simulink model "Case3_IEEE39_UGFLandGFM_2022b"  (R2022b)
settings: Solver=VariableStepAuto  StartTime=0.0  StopTime=30  RelTol=1e-3
InitFcn:
  | IEEE39data_UGFLandGFM;
undefined symbols (not defined in the file): Fref, IBR, line, Sbase, SG, UGFML, Vbase
libraries: spsThreePhaseVIMeasurementLib x66, spsThreePhasePISectionLineLib x35, spsPLL3phLib x25, spsControlledVoltageSourceLib x21, spsThreePhaseParallelRLCLoadLib x21, powerlib_extras x20, spsGroundLib x20, spsMeanLib x20, spsRMSLib x15, spsabctodq0Lib x11, spsThreePhaseSeriesRLCBranchLib x10, slpidlib x10
(part 3 of 5)

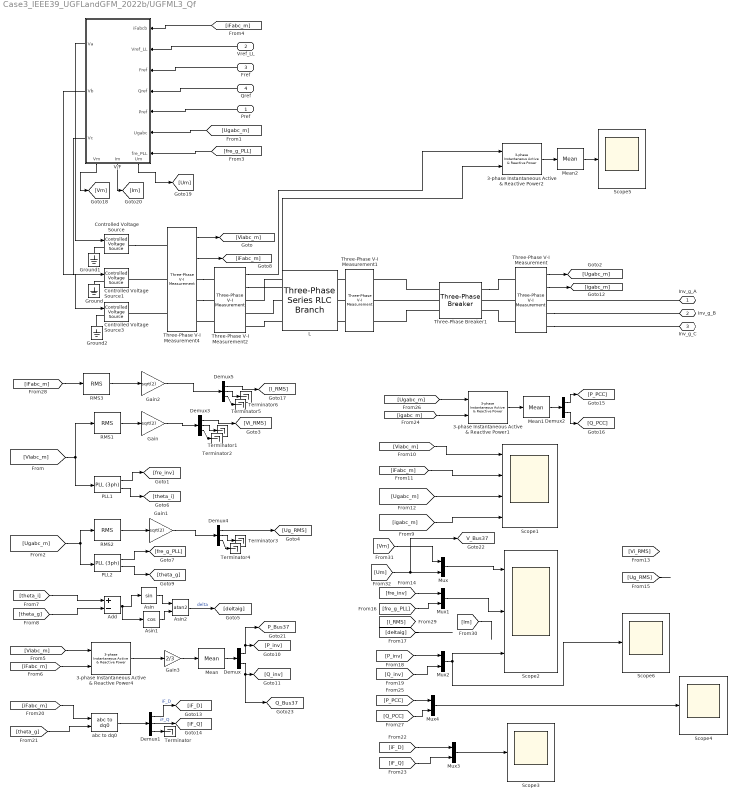
== system Case3_IEEE39_UGFLandGFM_2022b/UGFML3_Qf ==
  Pref : Inport
  Vref_LL : Inport  Port=2
  Fref : Inport  Port=3
  Qref : Inport  Port=4
  3-phase Instantaneous Active & Reactive Power1 : powerlib_extras/Measurements/3-phase  Instantaneous  Active & Reactive Power
  3-phase Instantaneous Active & Reactive Power2 : powerlib_extras/Measurements/3-phase  Instantaneous  Active & Reactive Power
  3-phase Instantaneous Active & Reactive Power4 : powerlib_extras/Measurements/3-phase  Instantaneous  Active & Reactive Power
  Add : Sum  Inputs=+-
  Asin : Trigonometry
  Asin1 : Trigonometry  Operator=cos
  Asin2 : Trigonometry  Operator=atan2
  Controlled Voltage Source : spsControlledVoltageSourceLib/Controlled Voltage Source  Initialize=on  Source_Type=DC  Amplitude=300  Phase=0  Frequency=60  Measurements=None
  Controlled Voltage Source1 : spsControlledVoltageSourceLib/Controlled Voltage Source  Initialize=on  Source_Type=DC  Amplitude=300  Phase=-120  Frequency=60  Measurements=None
  Controlled Voltage Source3 : spsControlledVoltageSourceLib/Controlled Voltage Source  Initialize=on  Source_Type=DC  Amplitude=300  Phase=120  Frequency=60  Measurements=None
  Demux : Demux  Outputs=2
  Demux{1,3..5} (4 alike) : Demux  Outputs=3
  Demux2 : Demux  Outputs=2
  Gain : Gain  Gain=sqrt(2)
  Gain1 : Gain  Gain=sqrt(2)
  Gain2 : Gain  Gain=sqrt(2)
  Gain3 : Gain  Gain=2/3
  Ground : spsGroundLib/Ground  LConnTagsString=a
  Ground1 : spsGroundLib/Ground  LConnTagsString=a
  Ground2 : spsGroundLib/Ground  LConnTagsString=a
  L : spsThreePhaseSeriesRLCBranchLib/Three-Phase Series RLC Branch  LConnTagsString=A|B|C  RConnTagsString=A|B|C  BranchType=RL  Resistance=0.01*Vbase^2/Sbase  Inductance=0.05*(Vbase^2/Sbase/377)  Capacitance=1.0  Measurements=None
  Mean : spsMeanLib/Mean  Freq=60  Vinit=0  Ts=5e-4
  Mean1 : spsMeanLib/Mean  Freq=60  Vinit=0  Ts=1e-4
  Mean2 : spsMeanLib/Mean  Freq=60  Vinit=0  Ts=5e-4
  Mux{,1..4} (5 alike) : Mux  Inputs=2
  PLL1 : spsPLL3phLib/PLL (3ph)  Fmin=35  Par_Init=[0, 60]  ParK=[180, 3200, 1]  TcD=1e-4  MaxRateChangeFreq=12  FilterCutOffFreq=25  Ts=1e-5  AGC=on
  PLL2 : spsPLL3phLib/PLL (3ph)  Fmin=35  Par_Init=[0, 60]  ParK=[180, 3200, 1]  TcD=1e-4  MaxRateChangeFreq=12  FilterCutOffFreq=25  Ts=1e-5  AGC=on
  RMS1 : spsRMSLib/RMS  TrueRMS=on  Freq=60  RMSInit=1  Ts=1e-4
  RMS2 : spsRMSLib/RMS  TrueRMS=on  Freq=60  RMSInit=1  Ts=1e-4
  RMS3 : spsRMSLib/RMS  TrueRMS=on  Freq=60  RMSInit=1  Ts=5e-4
  Scope1 : Scope  NumInputPorts=4
  Scope2 : Scope  NumInputPorts=3
  Scope{3..6} (4 alike) : Scope
  Terminator{,1..6} (7 alike) : Terminator
  Three-Phase V-I Measurement : spsThreePhaseVIMeasurementLib/Three-Phase V-I Measurement  VoltageMeasurement=phase-to-ground  SetLabelV=off  LabelV=Vabc  Vpu=on  VpuLL=off  CurrentMeasurement=yes  SetLabelI=off  LabelI=Iabc  Ipu=on  Pbase=Sbase  Vbase=Vbase  OutputType=Complex  PhasorSimulation=off  PSBequivalent=0
  Three-Phase V-I Measurement1 : spsThreePhaseVIMeasurementLib/Three-Phase V-I Measurement  VoltageMeasurement=no  SetLabelV=off  LabelV=Vabc  Vpu=off  VpuLL=off  CurrentMeasurement=no  SetLabelI=off  LabelI=Iabc  Ipu=off  Pbase=1e5  Vbase=380  OutputType=Complex  PhasorSimulation=off  PSBequivalent=0
  Three-Phase V-I Measurement2 : spsThreePhaseVIMeasurementLib/Three-Phase V-I Measurement  VoltageMeasurement=phase-to-ground  SetLabelV=off  LabelV=Vabc  Vpu=off  VpuLL=off  CurrentMeasurement=yes  SetLabelI=off  LabelI=Iabc  Ipu=off  Pbase=Sbase  Vbase=Vbase  OutputType=Complex  PhasorSimulation=off  PSBequivalent=0
  Three-Phase V-I Measurement4 : spsThreePhaseVIMeasurementLib/Three-Phase V-I Measurement  VoltageMeasurement=phase-to-ground  SetLabelV=off  LabelV=u  Vpu=on  VpuLL=off  CurrentMeasurement=yes  SetLabelI=off  LabelI=iFabcp3  Ipu=on  Pbase=Sbase  Vbase=Vbase  OutputType=Complex  PhasorSimulation=off  PSBequivalent=0
  Three-Phase Breaker1 : spsThreePhaseBreakerLib/Three-Phase Breaker  InitialState=open  SwitchA=on  SwitchB=on  SwitchC=on  SwitchTimes=[0.1]  External=off  BreakerResistance=0.0001  SnubberResistance=1e8  SnubberCapacitance=inf  Measurements=None
  V/F : Subsystem
      settings: PortSchema="{\"entries\":[{\"content\":{\"sides\":[{\"content\":{\"connectorIds\":[\"In1\",\"In2\",\"In3\",\"In4\",\"In5\",\"In6\",\"In7\"]},\"type\":\"ConnectorPlacement.EquallySpacedRectSide\",\"uuid\":\"ccc7dc11-36db-4369-953c-0655fd1e2442\"},{\"content\":{\"connectorIds\":[\"Out1\",\"Out2\",\"Out3\"],\"side\":\"RIGHT\"},\"type\":\"ConnectorPlacement.EquallySpacedRectSide\",\"uuid\":\"5735cf9b-d8e4-4bce-b2db-12738d0d9e4d\"},{\"content\":{\"side\":\"TOP\"},\"type\":\"ConnectorPlacement.EquallySpacedRectSide\",\"uuid\":\"e010782d-2644-4ebf-978f-8395ad947d0e\"},{\"content\":{\"connectorIds\":[\"Out4\",\"Out5\",\"Out6\"],\"side\":\"BOTTOM\"},\"type\":\"ConnectorPlacement.EquallySpacedRectSide\",\"uuid\":\"5965ef6f-6121-4d63-9a5a-1f7a3d153058\"}]},\"type\":\"ConnectorPlacement.EquallySpacedConnector\",\"uuid\":\"be33ea6e-20ef-4fc3-81eb-341d11cc9c18\"}],\"packageUris\":[\"http://schema.mathworks.com/mf0/Connector/R2020b\"],\"version\":\"1.0\"}"
  abc to dq0 : spsabctodq0Lib/abc to dq0  Alignment=90 degrees behind phase A axis
  Inv_g_A : PMIOPort  Side=Right
  Inv_g_B : PMIOPort  Port=2  Side=Right
  Inv_g_C : PMIOPort  Port=3  Side=Right
  tag scope: P_Bus37=global, Q_Bus37=global, V_Bus37=global
  wires:
  Three-Phase V-I Measurement/1 -> [Ugabc_m]
  Vref_LL/1 -> V/F/2(Vref_LL)
  V/F/2(Vb) -> Controlled Voltage Source1/1
  V/F/3(Vc) -> Controlled Voltage Source3/1
  Pref/1 -> V/F/5(Pref)
  Qref/1 -> V/F/4(Qref)
  Fref/1 -> V/F/3(Fref)
  RMS1/1 -> Gain/1
  Three-Phase V-I Measurement4/1 -> [Viabc_m]
  [Viabc_m] -> RMS1/1, PLL1/1
  PLL1/2 -> [theta_i]
  PLL1/1 -> [fre_inv]
  [Ugabc_m] -> V/F/6(Ugabc)
  [Ugabc_m] -> PLL2/1, RMS2/1
  RMS2/1 -> Gain1/1
  PLL2/2 -> [theta_g]
  PLL2/1 -> [fre_g_PLL]
  Three-Phase V-I Measurement4/2 -> [iFabc_m]
  [iFabc_m] -> V/F/1(iFabcb)
  [Viabc_m] -> 3-phase Instantaneous Active & Reactive Power4/1
  [iFabc_m] -> 3-phase Instantaneous Active & Reactive Power4/2
  Mean/1 -> Demux/1
  Demux/1 -> [P_Bus37], [P_inv]
  Demux/2 -> [Q_Bus37], [Q_inv]
  Three-Phase V-I Measurement/2 -> [igabc_m]
  [Viabc_m] -> Scope1/1
  [iFabc_m] -> Scope1/2
  [Ugabc_m] -> Scope1/3
  [igabc_m] -> Scope1/4
  [fre_inv] -> Mux1/1
  [Ug_RMS] -> ?
  Mux/1 -> Scope2/1
  [fre_g_PLL] -> Mux1/2
  Mux1/1 -> Scope2/2
  [deltaig] -> ?
  [P_inv] -> Mux2/1
  [Q_inv] -> Mux2/2
  Mux2/1 -> Scope2/3, Scope6/1
  Gain/1 -> Demux3/1
  [fre_g_PLL] -> V/F/7(fre_PLL)
  [theta_i] -> Add/1
  Add/1 -> Asin/1, Asin1/1
  [theta_g] -> Add/2
  Asin/1 -> Asin2/1
  Asin1/1 -> Asin2/2
  Asin2/1 -> [deltaig]  "delta"
  [iFabc_m] -> abc to dq0/1
  [theta_g] -> abc to dq0/2
  abc to dq0/1 -> Demux1/1
  Demux1/3 -> Terminator/1
  Demux1/1 -> [iF_D]  "iF_D"
  Demux1/2 -> [iF_Q]  "iF_Q"
  [iF_D] -> Mux3/1
  [iF_Q] -> Mux3/2
  Mux3/1 -> Scope3/1
  V/F/1(Va) -> Controlled Voltage Source/1
  Demux2/2 -> [Q_PCC]
  [Ugabc_m] -> 3-phase Instantaneous Active & Reactive Power1/1
  [igabc_m] -> 3-phase Instantaneous Active & Reactive Power1/2
  Mean1/1 -> Demux2/1
  Demux2/1 -> [P_PCC]
  3-phase Instantaneous Active & Reactive Power1/1 -> Mean1/1
  [P_PCC] -> Mux4/1
  [Q_PCC] -> Mux4/2
  Mux4/1 -> Scope4/1
  Demux3/1 -> [Vi_RMS]
  Demux3/2 -> Terminator1/1
  Demux3/3 -> Terminator2/1
  Demux4/3 -> Terminator4/1
  Demux4/1 -> [Ug_RMS]
  Demux4/2 -> Terminator3/1
  Gain1/1 -> Demux4/1
  [iFabc_m] -> RMS3/1
  RMS3/1 -> Gain2/1
  Demux5/3 -> Terminator6/1
  Demux5/1 -> [I_RMS]
  Demux5/2 -> Terminator5/1
  Gain2/1 -> Demux5/1
  Three-Phase V-I Measurement2/1 -> 3-phase Instantaneous Active & Reactive Power2/1
  Mean2/1 -> Scope5/1
  Three-Phase V-I Measurement2/2 -> 3-phase Instantaneous Active & Reactive Power2/2
  3-phase Instantaneous Active & Reactive Power2/1 -> Mean2/1
  Gain3/1 -> Mean/1
  3-phase Instantaneous Active & Reactive Power4/1 -> Gain3/1
  [Vm] -> Mux/1
  [Um] -> [V_Bus37], Mux/2
  [Im] -> ?
  V/F/5(Im) -> [Im]
  V/F/6(Vm) -> [Vm]
  V/F/4(Um) -> [Um]
  connections:
  Three-Phase V-I Measurement/RConn2 -- Inv_g_B/RConn1
  Three-Phase V-I Measurement4/LConn2 -- Controlled Voltage Source1/RConn1
  Controlled Voltage Source/RConn1 -- Three-Phase V-I Measurement4/LConn1
  Three-Phase V-I Measurement4/LConn3 -- Controlled Voltage Source3/RConn1
  Three-Phase Breaker1/LConn3 -- Three-Phase V-I Measurement1/RConn3
  Three-Phase V-I Measurement/RConn3 -- Inv_g_C/RConn1
  Inv_g_A/RConn1 -- Three-Phase V-I Measurement/RConn1
  Three-Phase V-I Measurement4/RConn1 -- Three-Phase V-I Measurement2/LConn1
  Three-Phase V-I Measurement4/RConn2 -- Three-Phase V-I Measurement2/LConn2
  Three-Phase V-I Measurement2/LConn3 -- Three-Phase V-I Measurement4/RConn3
  Controlled Voltage Source1/LConn1 -- Ground/LConn1
  Three-Phase Breaker1/LConn2 -- Three-Phase V-I Measurement1/RConn2
  Three-Phase Breaker1/LConn1 -- Three-Phase V-I Measurement1/RConn1
  Three-Phase V-I Measurement1/LConn1 -- L/RConn1
  Three-Phase V-I Measurement1/LConn2 -- L/RConn2
  Three-Phase V-I Measurement1/LConn3 -- L/RConn3
  Controlled Voltage Source/LConn1 -- Ground1/LConn1
  Controlled Voltage Source3/LConn1 -- Ground2/LConn1
  Three-Phase Breaker1/RConn1 -- Three-Phase V-I Measurement/LConn1
  Three-Phase V-I Measurement/LConn2 -- Three-Phase Breaker1/RConn2
  Three-Phase V-I Measurement/LConn3 -- Three-Phase Breaker1/RConn3
  L/LConn1 -- Three-Phase V-I Measurement2/RConn1
  L/LConn2 -- Three-Phase V-I Measurement2/RConn2
  L/LConn3 -- Three-Phase V-I Measurement2/RConn3

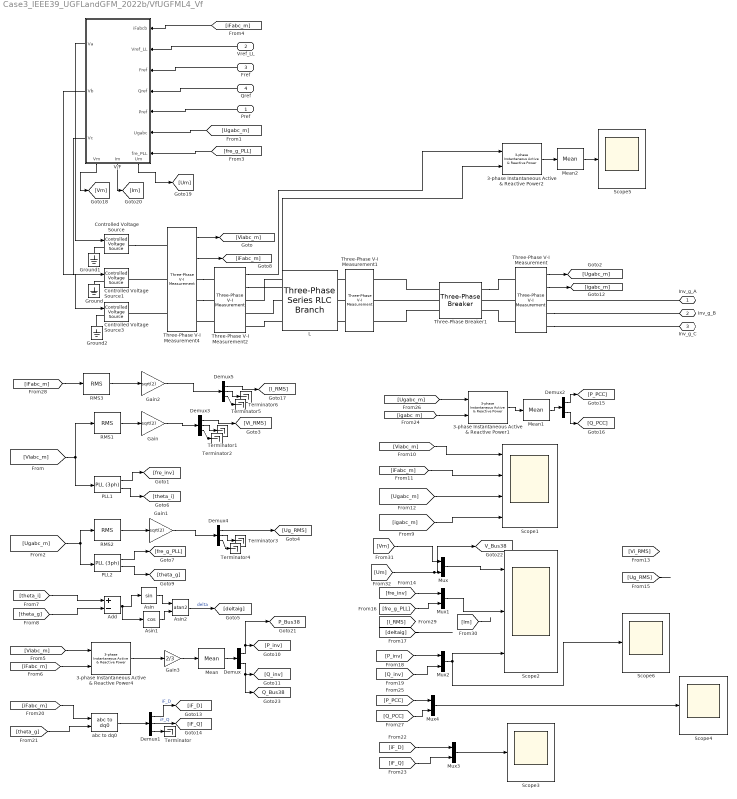
== system Case3_IEEE39_UGFLandGFM_2022b/VfUGFML4_Vf ==
  Pref : Inport
  Vref_LL : Inport  Port=2
  Fref : Inport  Port=3
  Qref : Inport  Port=4
  3-phase Instantaneous Active & Reactive Power1 : powerlib_extras/Measurements/3-phase  Instantaneous  Active & Reactive Power
  3-phase Instantaneous Active & Reactive Power2 : powerlib_extras/Measurements/3-phase  Instantaneous  Active & Reactive Power
  3-phase Instantaneous Active & Reactive Power4 : powerlib_extras/Measurements/3-phase  Instantaneous  Active & Reactive Power
  Add : Sum  Inputs=+-
  Asin : Trigonometry
  Asin1 : Trigonometry  Operator=cos
  Asin2 : Trigonometry  Operator=atan2
  Controlled Voltage Source : spsControlledVoltageSourceLib/Controlled Voltage Source  Initialize=on  Source_Type=DC  Amplitude=300  Phase=0  Frequency=60  Measurements=None
  Controlled Voltage Source1 : spsControlledVoltageSourceLib/Controlled Voltage Source  Initialize=on  Source_Type=DC  Amplitude=300  Phase=-120  Frequency=60  Measurements=None
  Controlled Voltage Source3 : spsControlledVoltageSourceLib/Controlled Voltage Source  Initialize=on  Source_Type=DC  Amplitude=300  Phase=120  Frequency=60  Measurements=None
  Demux : Demux  Outputs=2
  Demux{1,3..5} (4 alike) : Demux  Outputs=3
  Demux2 : Demux  Outputs=2
  Gain : Gain  Gain=sqrt(2)
  Gain1 : Gain  Gain=sqrt(2)
  Gain2 : Gain  Gain=sqrt(2)
  Gain3 : Gain  Gain=2/3
  Ground : spsGroundLib/Ground  LConnTagsString=a
  Ground1 : spsGroundLib/Ground  LConnTagsString=a
  Ground2 : spsGroundLib/Ground  LConnTagsString=a
  L : spsThreePhaseSeriesRLCBranchLib/Three-Phase Series RLC Branch  LConnTagsString=A|B|C  RConnTagsString=A|B|C  BranchType=RL  Resistance=0.01*Vbase^2/Sbase  Inductance=0.05*(Vbase^2/Sbase/377)  Capacitance=1.0  Measurements=None
  Mean : spsMeanLib/Mean  Freq=60  Vinit=0  Ts=5e-4
  Mean1 : spsMeanLib/Mean  Freq=60  Vinit=0  Ts=1e-4
  Mean2 : spsMeanLib/Mean  Freq=60  Vinit=0  Ts=5e-4
  Mux{,1..4} (5 alike) : Mux  Inputs=2
  PLL1 : spsPLL3phLib/PLL (3ph)  Fmin=35  Par_Init=[0, 60]  ParK=[180, 3200, 1]  TcD=1e-4  MaxRateChangeFreq=12  FilterCutOffFreq=25  Ts=1e-5  AGC=on
  PLL2 : spsPLL3phLib/PLL (3ph)  Fmin=35  Par_Init=[0, 60]  ParK=[180, 3200, 1]  TcD=1e-4  MaxRateChangeFreq=12  FilterCutOffFreq=25  Ts=1e-5  AGC=on
  RMS1 : spsRMSLib/RMS  TrueRMS=on  Freq=60  RMSInit=1  Ts=1e-4
  RMS2 : spsRMSLib/RMS  TrueRMS=on  Freq=60  RMSInit=1  Ts=1e-4
  RMS3 : spsRMSLib/RMS  TrueRMS=on  Freq=60  RMSInit=1  Ts=5e-4
  Scope1 : Scope  NumInputPorts=4
  Scope2 : Scope  NumInputPorts=3
  Scope{3..6} (4 alike) : Scope
  Terminator{,1..6} (7 alike) : Terminator
  Three-Phase V-I Measurement : spsThreePhaseVIMeasurementLib/Three-Phase V-I Measurement  VoltageMeasurement=phase-to-ground  SetLabelV=off  LabelV=Vabc  Vpu=on  VpuLL=off  CurrentMeasurement=yes  SetLabelI=off  LabelI=Iabc  Ipu=on  Pbase=Sbase  Vbase=Vbase  OutputType=Complex  PhasorSimulation=off  PSBequivalent=0
  Three-Phase V-I Measurement1 : spsThreePhaseVIMeasurementLib/Three-Phase V-I Measurement  VoltageMeasurement=no  SetLabelV=off  LabelV=Vabc  Vpu=off  VpuLL=off  CurrentMeasurement=no  SetLabelI=off  LabelI=Iabc  Ipu=off  Pbase=1e5  Vbase=380  OutputType=Complex  PhasorSimulation=off  PSBequivalent=0
  Three-Phase V-I Measurement2 : spsThreePhaseVIMeasurementLib/Three-Phase V-I Measurement  VoltageMeasurement=phase-to-ground  SetLabelV=off  LabelV=Vabc  Vpu=off  VpuLL=off  CurrentMeasurement=yes  SetLabelI=off  LabelI=Iabc  Ipu=off  Pbase=Sbase  Vbase=Vbase  OutputType=Complex  PhasorSimulation=off  PSBequivalent=0
  Three-Phase V-I Measurement4 : spsThreePhaseVIMeasurementLib/Three-Phase V-I Measurement  VoltageMeasurement=phase-to-ground  SetLabelV=off  LabelV=u  Vpu=on  VpuLL=off  CurrentMeasurement=yes  SetLabelI=off  LabelI=iFabcp3  Ipu=on  Pbase=Sbase  Vbase=Vbase  OutputType=Complex  PhasorSimulation=off  PSBequivalent=0
  Three-Phase Breaker1 : spsThreePhaseBreakerLib/Three-Phase Breaker  InitialState=open  SwitchA=on  SwitchB=on  SwitchC=on  SwitchTimes=[0.1]  External=off  BreakerResistance=0.0001  SnubberResistance=1e8  SnubberCapacitance=inf  Measurements=None
  V/F : Subsystem
      settings: PortSchema="{\"entries\":[{\"content\":{\"sides\":[{\"content\":{\"connectorIds\":[\"In1\",\"In2\",\"In3\",\"In4\",\"In5\",\"In6\",\"In7\"]},\"type\":\"ConnectorPlacement.EquallySpacedRectSide\",\"uuid\":\"ccc7dc11-36db-4369-953c-0655fd1e2442\"},{\"content\":{\"connectorIds\":[\"Out1\",\"Out2\",\"Out3\"],\"side\":\"RIGHT\"},\"type\":\"ConnectorPlacement.EquallySpacedRectSide\",\"uuid\":\"5735cf9b-d8e4-4bce-b2db-12738d0d9e4d\"},{\"content\":{\"side\":\"TOP\"},\"type\":\"ConnectorPlacement.EquallySpacedRectSide\",\"uuid\":\"e010782d-2644-4ebf-978f-8395ad947d0e\"},{\"content\":{\"connectorIds\":[\"Out4\",\"Out5\",\"Out6\"],\"side\":\"BOTTOM\"},\"type\":\"ConnectorPlacement.EquallySpacedRectSide\",\"uuid\":\"5965ef6f-6121-4d63-9a5a-1f7a3d153058\"}]},\"type\":\"ConnectorPlacement.EquallySpacedConnector\",\"uuid\":\"be33ea6e-20ef-4fc3-81eb-341d11cc9c18\"}],\"packageUris\":[\"http://schema.mathworks.com/mf0/Connector/R2020b\"],\"version\":\"1.0\"}"
  abc to dq0 : spsabctodq0Lib/abc to dq0  Alignment=90 degrees behind phase A axis
  Inv_g_A : PMIOPort  Side=Right
  Inv_g_B : PMIOPort  Port=2  Side=Right
  Inv_g_C : PMIOPort  Port=3  Side=Right
  tag scope: P_Bus38=global, Q_Bus38=global, V_Bus38=global
  wires:
  Three-Phase V-I Measurement/1 -> [Ugabc_m]
  Vref_LL/1 -> V/F/2(Vref_LL)
  V/F/2(Vb) -> Controlled Voltage Source1/1
  V/F/3(Vc) -> Controlled Voltage Source3/1
  Pref/1 -> V/F/5(Pref)
  Qref/1 -> V/F/4(Qref)
  Fref/1 -> V/F/3(Fref)
  RMS1/1 -> Gain/1
  Three-Phase V-I Measurement4/1 -> [Viabc_m]
  [Viabc_m] -> RMS1/1, PLL1/1
  PLL1/2 -> [theta_i]
  PLL1/1 -> [fre_inv]
  [Ugabc_m] -> V/F/6(Ugabc)
  [Ugabc_m] -> PLL2/1, RMS2/1
  RMS2/1 -> Gain1/1
  PLL2/2 -> [theta_g]
  PLL2/1 -> [fre_g_PLL]
  Three-Phase V-I Measurement4/2 -> [iFabc_m]
  [iFabc_m] -> V/F/1(iFabcb)
  [Viabc_m] -> 3-phase Instantaneous Active & Reactive Power4/1
  [iFabc_m] -> 3-phase Instantaneous Active & Reactive Power4/2
  Mean/1 -> Demux/1
  Demux/1 -> [P_Bus38], [P_inv]
  Demux/2 -> [Q_Bus38], [Q_inv]
  Three-Phase V-I Measurement/2 -> [igabc_m]
  [Viabc_m] -> Scope1/1
  [iFabc_m] -> Scope1/2
  [Ugabc_m] -> Scope1/3
  [igabc_m] -> Scope1/4
  [fre_inv] -> Mux1/1
  [Ug_RMS] -> ?
  Mux/1 -> Scope2/1
  [fre_g_PLL] -> Mux1/2
  Mux1/1 -> Scope2/2
  [deltaig] -> ?
  [P_inv] -> Mux2/1
  [Q_inv] -> Mux2/2
  Mux2/1 -> Scope2/3, Scope6/1
  Gain/1 -> Demux3/1
  [fre_g_PLL] -> V/F/7(fre_PLL)
  [theta_i] -> Add/1
  Add/1 -> Asin/1, Asin1/1
  [theta_g] -> Add/2
  Asin/1 -> Asin2/1
  Asin1/1 -> Asin2/2
  Asin2/1 -> [deltaig]  "delta"
  [iFabc_m] -> abc to dq0/1
  [theta_g] -> abc to dq0/2
  abc to dq0/1 -> Demux1/1
  Demux1/3 -> Terminator/1
  Demux1/1 -> [iF_D]  "iF_D"
  Demux1/2 -> [iF_Q]  "iF_Q"
  [iF_D] -> Mux3/1
  [iF_Q] -> Mux3/2
  Mux3/1 -> Scope3/1
  V/F/1(Va) -> Controlled Voltage Source/1
  Demux2/2 -> [Q_PCC]
  [Ugabc_m] -> 3-phase Instantaneous Active & Reactive Power1/1
  [igabc_m] -> 3-phase Instantaneous Active & Reactive Power1/2
  Mean1/1 -> Demux2/1
  Demux2/1 -> [P_PCC]
  3-phase Instantaneous Active & Reactive Power1/1 -> Mean1/1
  [P_PCC] -> Mux4/1
  [Q_PCC] -> Mux4/2
  Mux4/1 -> Scope4/1
  Demux3/1 -> [Vi_RMS]
  Demux3/2 -> Terminator1/1
  Demux3/3 -> Terminator2/1
  Demux4/3 -> Terminator4/1
  Demux4/1 -> [Ug_RMS]
  Demux4/2 -> Terminator3/1
  Gain1/1 -> Demux4/1
  [iFabc_m] -> RMS3/1
  RMS3/1 -> Gain2/1
  Demux5/3 -> Terminator6/1
  Demux5/1 -> [I_RMS]
  Demux5/2 -> Terminator5/1
  Gain2/1 -> Demux5/1
  Three-Phase V-I Measurement2/1 -> 3-phase Instantaneous Active & Reactive Power2/1
  Mean2/1 -> Scope5/1
  Three-Phase V-I Measurement2/2 -> 3-phase Instantaneous Active & Reactive Power2/2
  3-phase Instantaneous Active & Reactive Power2/1 -> Mean2/1
  Gain3/1 -> Mean/1
  3-phase Instantaneous Active & Reactive Power4/1 -> Gain3/1
  [Vm] -> Mux/1
  [Um] -> [V_Bus38], Mux/2
  [Im] -> ?
  V/F/5(Im) -> [Im]
  V/F/6(Vm) -> [Vm]
  V/F/4(Um) -> [Um]
  connections:
  Three-Phase V-I Measurement/RConn2 -- Inv_g_B/RConn1
  Three-Phase V-I Measurement4/LConn2 -- Controlled Voltage Source1/RConn1
  Controlled Voltage Source/RConn1 -- Three-Phase V-I Measurement4/LConn1
  Three-Phase V-I Measurement4/LConn3 -- Controlled Voltage Source3/RConn1
  Three-Phase Breaker1/LConn3 -- Three-Phase V-I Measurement1/RConn3
  Three-Phase V-I Measurement/RConn3 -- Inv_g_C/RConn1
  Inv_g_A/RConn1 -- Three-Phase V-I Measurement/RConn1
  Three-Phase V-I Measurement4/RConn1 -- Three-Phase V-I Measurement2/LConn1
  Three-Phase V-I Measurement4/RConn2 -- Three-Phase V-I Measurement2/LConn2
  Three-Phase V-I Measurement2/LConn3 -- Three-Phase V-I Measurement4/RConn3
  Controlled Voltage Source1/LConn1 -- Ground/LConn1
  Three-Phase Breaker1/LConn2 -- Three-Phase V-I Measurement1/RConn2
  Three-Phase Breaker1/LConn1 -- Three-Phase V-I Measurement1/RConn1
  Three-Phase V-I Measurement1/LConn1 -- L/RConn1
  Three-Phase V-I Measurement1/LConn2 -- L/RConn2
  Three-Phase V-I Measurement1/LConn3 -- L/RConn3
  Controlled Voltage Source/LConn1 -- Ground1/LConn1
  Controlled Voltage Source3/LConn1 -- Ground2/LConn1
  Three-Phase Breaker1/RConn1 -- Three-Phase V-I Measurement/LConn1
  Three-Phase V-I Measurement/LConn2 -- Three-Phase Breaker1/RConn2
  Three-Phase V-I Measurement/LConn3 -- Three-Phase Breaker1/RConn3
  L/LConn1 -- Three-Phase V-I Measurement2/RConn1
  L/LConn2 -- Three-Phase V-I Measurement2/RConn2
  L/LConn3 -- Three-Phase V-I Measurement2/RConn3

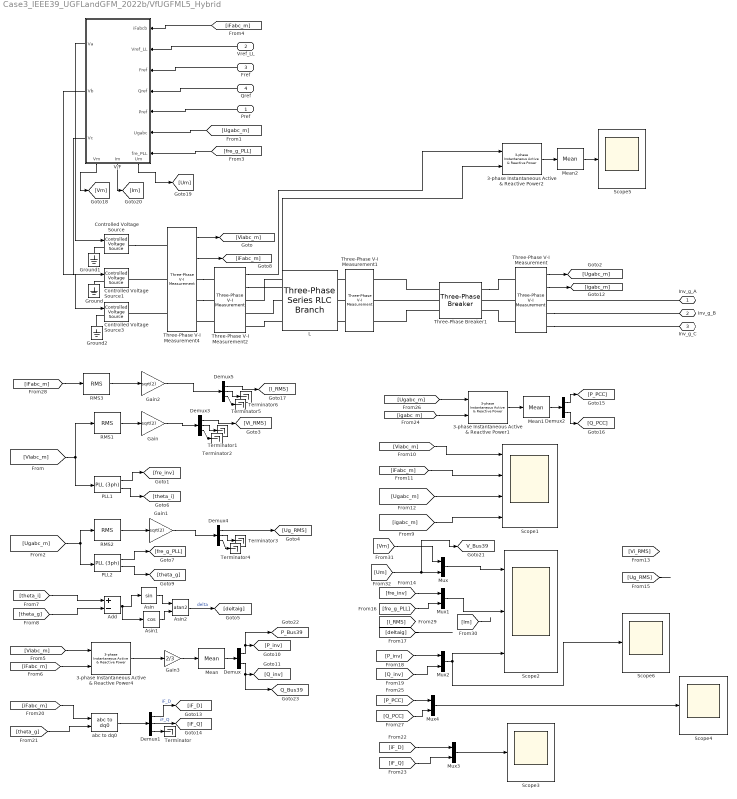
== system Case3_IEEE39_UGFLandGFM_2022b/VfUGFML5_Hybrid ==
  Pref : Inport
  Vref_LL : Inport  Port=2
  Fref : Inport  Port=3
  Qref : Inport  Port=4
  3-phase Instantaneous Active & Reactive Power1 : powerlib_extras/Measurements/3-phase  Instantaneous  Active & Reactive Power
  3-phase Instantaneous Active & Reactive Power2 : powerlib_extras/Measurements/3-phase  Instantaneous  Active & Reactive Power
  3-phase Instantaneous Active & Reactive Power4 : powerlib_extras/Measurements/3-phase  Instantaneous  Active & Reactive Power
  Add : Sum  Inputs=+-
  Asin : Trigonometry
  Asin1 : Trigonometry  Operator=cos
  Asin2 : Trigonometry  Operator=atan2
  Controlled Voltage Source : spsControlledVoltageSourceLib/Controlled Voltage Source  Initialize=on  Source_Type=DC  Amplitude=300  Phase=0  Frequency=60  Measurements=None
  Controlled Voltage Source1 : spsControlledVoltageSourceLib/Controlled Voltage Source  Initialize=on  Source_Type=DC  Amplitude=300  Phase=-120  Frequency=60  Measurements=None
  Controlled Voltage Source3 : spsControlledVoltageSourceLib/Controlled Voltage Source  Initialize=on  Source_Type=DC  Amplitude=300  Phase=120  Frequency=60  Measurements=None
  Demux : Demux  Outputs=2
  Demux{1,3..5} (4 alike) : Demux  Outputs=3
  Demux2 : Demux  Outputs=2
  Gain : Gain  Gain=sqrt(2)
  Gain1 : Gain  Gain=sqrt(2)
  Gain2 : Gain  Gain=sqrt(2)
  Gain3 : Gain  Gain=2/3
  Ground : spsGroundLib/Ground  LConnTagsString=a
  Ground1 : spsGroundLib/Ground  LConnTagsString=a
  Ground2 : spsGroundLib/Ground  LConnTagsString=a
  L : spsThreePhaseSeriesRLCBranchLib/Three-Phase Series RLC Branch  LConnTagsString=A|B|C  RConnTagsString=A|B|C  BranchType=RL  Resistance=0.01*Vbase^2/Sbase  Inductance=0.05*(Vbase^2/Sbase/377)  Capacitance=1.0  Measurements=None
  Mean : spsMeanLib/Mean  Freq=60  Vinit=0  Ts=5e-4
  Mean1 : spsMeanLib/Mean  Freq=60  Vinit=0  Ts=1e-4
  Mean2 : spsMeanLib/Mean  Freq=60  Vinit=0  Ts=5e-4
  Mux{,1..4} (5 alike) : Mux  Inputs=2
  PLL1 : spsPLL3phLib/PLL (3ph)  Fmin=35  Par_Init=[0, 60]  ParK=[180, 3200, 1]  TcD=1e-4  MaxRateChangeFreq=12  FilterCutOffFreq=25  Ts=1e-5  AGC=on
  PLL2 : spsPLL3phLib/PLL (3ph)  Fmin=35  Par_Init=[0, 60]  ParK=[180, 3200, 1]  TcD=1e-4  MaxRateChangeFreq=12  FilterCutOffFreq=25  Ts=1e-5  AGC=on
  RMS1 : spsRMSLib/RMS  TrueRMS=on  Freq=60  RMSInit=1  Ts=1e-4
  RMS2 : spsRMSLib/RMS  TrueRMS=on  Freq=60  RMSInit=1  Ts=1e-4
  RMS3 : spsRMSLib/RMS  TrueRMS=on  Freq=60  RMSInit=1  Ts=5e-4
  Scope1 : Scope  NumInputPorts=4
  Scope2 : Scope  NumInputPorts=3
  Scope{3..6} (4 alike) : Scope
  Terminator{,1..6} (7 alike) : Terminator
  Three-Phase V-I Measurement : spsThreePhaseVIMeasurementLib/Three-Phase V-I Measurement  VoltageMeasurement=phase-to-ground  SetLabelV=off  LabelV=Vabc  Vpu=on  VpuLL=off  CurrentMeasurement=yes  SetLabelI=off  LabelI=Iabc  Ipu=on  Pbase=Sbase  Vbase=Vbase  OutputType=Complex  PhasorSimulation=off  PSBequivalent=0
  Three-Phase V-I Measurement1 : spsThreePhaseVIMeasurementLib/Three-Phase V-I Measurement  VoltageMeasurement=no  SetLabelV=off  LabelV=Vabc  Vpu=off  VpuLL=off  CurrentMeasurement=no  SetLabelI=off  LabelI=Iabc  Ipu=off  Pbase=1e5  Vbase=380  OutputType=Complex  PhasorSimulation=off  PSBequivalent=0
  Three-Phase V-I Measurement2 : spsThreePhaseVIMeasurementLib/Three-Phase V-I Measurement  VoltageMeasurement=phase-to-ground  SetLabelV=off  LabelV=Vabc  Vpu=off  VpuLL=off  CurrentMeasurement=yes  SetLabelI=off  LabelI=Iabc  Ipu=off  Pbase=Sbase  Vbase=Vbase  OutputType=Complex  PhasorSimulation=off  PSBequivalent=0
  Three-Phase V-I Measurement4 : spsThreePhaseVIMeasurementLib/Three-Phase V-I Measurement  VoltageMeasurement=phase-to-ground  SetLabelV=off  LabelV=u  Vpu=on  VpuLL=off  CurrentMeasurement=yes  SetLabelI=off  LabelI=iFabcp3  Ipu=on  Pbase=Sbase  Vbase=Vbase  OutputType=Complex  PhasorSimulation=off  PSBequivalent=0
  Three-Phase Breaker1 : spsThreePhaseBreakerLib/Three-Phase Breaker  InitialState=open  SwitchA=on  SwitchB=on  SwitchC=on  SwitchTimes=[0.1]  External=off  BreakerResistance=0.0001  SnubberResistance=1e8  SnubberCapacitance=inf  Measurements=None
  V/F : Subsystem
      settings: PortSchema="{\"entries\":[{\"content\":{\"sides\":[{\"content\":{\"connectorIds\":[\"In1\",\"In2\",\"In3\",\"In4\",\"In5\",\"In6\",\"In7\"]},\"type\":\"ConnectorPlacement.EquallySpacedRectSide\",\"uuid\":\"ccc7dc11-36db-4369-953c-0655fd1e2442\"},{\"content\":{\"connectorIds\":[\"Out1\",\"Out2\",\"Out3\"],\"side\":\"RIGHT\"},\"type\":\"ConnectorPlacement.EquallySpacedRectSide\",\"uuid\":\"5735cf9b-d8e4-4bce-b2db-12738d0d9e4d\"},{\"content\":{\"side\":\"TOP\"},\"type\":\"ConnectorPlacement.EquallySpacedRectSide\",\"uuid\":\"e010782d-2644-4ebf-978f-8395ad947d0e\"},{\"content\":{\"connectorIds\":[\"Out4\",\"Out5\",\"Out6\"],\"side\":\"BOTTOM\"},\"type\":\"ConnectorPlacement.EquallySpacedRectSide\",\"uuid\":\"5965ef6f-6121-4d63-9a5a-1f7a3d153058\"}]},\"type\":\"ConnectorPlacement.EquallySpacedConnector\",\"uuid\":\"be33ea6e-20ef-4fc3-81eb-341d11cc9c18\"}],\"packageUris\":[\"http://schema.mathworks.com/mf0/Connector/R2020b\"],\"version\":\"1.0\"}"
  abc to dq0 : spsabctodq0Lib/abc to dq0  Alignment=90 degrees behind phase A axis
  Inv_g_A : PMIOPort  Side=Right
  Inv_g_B : PMIOPort  Port=2  Side=Right
  Inv_g_C : PMIOPort  Port=3  Side=Right
  tag scope: P_Bus39=global, Q_Bus39=global, V_Bus39=global
  wires:
  Three-Phase V-I Measurement/1 -> [Ugabc_m]
  Vref_LL/1 -> V/F/2(Vref_LL)
  V/F/2(Vb) -> Controlled Voltage Source1/1
  V/F/3(Vc) -> Controlled Voltage Source3/1
  Pref/1 -> V/F/5(Pref)
  Qref/1 -> V/F/4(Qref)
  Fref/1 -> V/F/3(Fref)
  RMS1/1 -> Gain/1
  Three-Phase V-I Measurement4/1 -> [Viabc_m]
  [Viabc_m] -> RMS1/1, PLL1/1
  PLL1/2 -> [theta_i]
  PLL1/1 -> [fre_inv]
  [Ugabc_m] -> V/F/6(Ugabc)
  [Ugabc_m] -> PLL2/1, RMS2/1
  RMS2/1 -> Gain1/1
  PLL2/2 -> [theta_g]
  PLL2/1 -> [fre_g_PLL]
  Three-Phase V-I Measurement4/2 -> [iFabc_m]
  [iFabc_m] -> V/F/1(iFabcb)
  [Viabc_m] -> 3-phase Instantaneous Active & Reactive Power4/1
  [iFabc_m] -> 3-phase Instantaneous Active & Reactive Power4/2
  Mean/1 -> Demux/1
  Demux/2 -> [Q_Bus39], [Q_inv]
  Three-Phase V-I Measurement/2 -> [igabc_m]
  [Viabc_m] -> Scope1/1
  [iFabc_m] -> Scope1/2
  [Ugabc_m] -> Scope1/3
  [igabc_m] -> Scope1/4
  [fre_inv] -> Mux1/1
  [Ug_RMS] -> ?
  Mux/1 -> Scope2/1
  [fre_g_PLL] -> Mux1/2
  Mux1/1 -> Scope2/2
  [deltaig] -> ?
  [P_inv] -> Mux2/1
  [Q_inv] -> Mux2/2
  Mux2/1 -> Scope2/3, Scope6/1
  Gain/1 -> Demux3/1
  [fre_g_PLL] -> V/F/7(fre_PLL)
  [theta_i] -> Add/1
  Add/1 -> Asin/1, Asin1/1
  [theta_g] -> Add/2
  Asin/1 -> Asin2/1
  Asin1/1 -> Asin2/2
  Asin2/1 -> [deltaig]  "delta"
  [iFabc_m] -> abc to dq0/1
  [theta_g] -> abc to dq0/2
  abc to dq0/1 -> Demux1/1
  Demux1/3 -> Terminator/1
  Demux1/1 -> [iF_D]  "iF_D"
  Demux1/2 -> [iF_Q]  "iF_Q"
  [iF_D] -> Mux3/1
  [iF_Q] -> Mux3/2
  Mux3/1 -> Scope3/1
  V/F/1(Va) -> Controlled Voltage Source/1
  Demux2/2 -> [Q_PCC]
  [Ugabc_m] -> 3-phase Instantaneous Active & Reactive Power1/1
  [igabc_m] -> 3-phase Instantaneous Active & Reactive Power1/2
  Mean1/1 -> Demux2/1
  Demux2/1 -> [P_PCC]
  3-phase Instantaneous Active & Reactive Power1/1 -> Mean1/1
  [P_PCC] -> Mux4/1
  [Q_PCC] -> Mux4/2
  Mux4/1 -> Scope4/1
  Demux3/1 -> [Vi_RMS]
  Demux3/2 -> Terminator1/1
  Demux3/3 -> Terminator2/1
  Demux4/3 -> Terminator4/1
  Demux4/1 -> [Ug_RMS]
  Demux4/2 -> Terminator3/1
  Gain1/1 -> Demux4/1
  [iFabc_m] -> RMS3/1
  RMS3/1 -> Gain2/1
  Demux5/3 -> Terminator6/1
  Demux5/1 -> [I_RMS]
  Demux5/2 -> Terminator5/1
  Gain2/1 -> Demux5/1
  Three-Phase V-I Measurement2/1 -> 3-phase Instantaneous Active & Reactive Power2/1
  Mean2/1 -> Scope5/1
  Three-Phase V-I Measurement2/2 -> 3-phase Instantaneous Active & Reactive Power2/2
  3-phase Instantaneous Active & Reactive Power2/1 -> Mean2/1
  Gain3/1 -> Mean/1
  3-phase Instantaneous Active & Reactive Power4/1 -> Gain3/1
  [Vm] -> Mux/1
  [Um] -> Mux/2, [V_Bus39]
  [Im] -> ?
  V/F/5(Im) -> [Im]
  V/F/6(Vm) -> [Vm]
  V/F/4(Um) -> [Um]
  Demux/1 -> [P_Bus39], [P_inv]
  connections:
  Three-Phase V-I Measurement/RConn2 -- Inv_g_B/RConn1
  Three-Phase V-I Measurement4/LConn2 -- Controlled Voltage Source1/RConn1
  Controlled Voltage Source/RConn1 -- Three-Phase V-I Measurement4/LConn1
  Three-Phase V-I Measurement4/LConn3 -- Controlled Voltage Source3/RConn1
  Three-Phase Breaker1/LConn3 -- Three-Phase V-I Measurement1/RConn3
  Three-Phase V-I Measurement/RConn3 -- Inv_g_C/RConn1
  Inv_g_A/RConn1 -- Three-Phase V-I Measurement/RConn1
  Three-Phase V-I Measurement4/RConn1 -- Three-Phase V-I Measurement2/LConn1
  Three-Phase V-I Measurement4/RConn2 -- Three-Phase V-I Measurement2/LConn2
  Three-Phase V-I Measurement2/LConn3 -- Three-Phase V-I Measurement4/RConn3
  Controlled Voltage Source1/LConn1 -- Ground/LConn1
  Three-Phase Breaker1/LConn2 -- Three-Phase V-I Measurement1/RConn2
  Three-Phase Breaker1/LConn1 -- Three-Phase V-I Measurement1/RConn1
  Three-Phase V-I Measurement1/LConn1 -- L/RConn1
  Three-Phase V-I Measurement1/LConn2 -- L/RConn2
  Three-Phase V-I Measurement1/LConn3 -- L/RConn3
  Controlled Voltage Source/LConn1 -- Ground1/LConn1
  Controlled Voltage Source3/LConn1 -- Ground2/LConn1
  Three-Phase Breaker1/RConn1 -- Three-Phase V-I Measurement/LConn1
  Three-Phase V-I Measurement/LConn2 -- Three-Phase Breaker1/RConn2
  Three-Phase V-I Measurement/LConn3 -- Three-Phase Breaker1/RConn3
  L/LConn1 -- Three-Phase V-I Measurement2/RConn1
  L/LConn2 -- Three-Phase V-I Measurement2/RConn2
  L/LConn3 -- Three-Phase V-I Measurement2/RConn3

== system Case3_IEEE39_UGFLandGFM_2022b/Bus voltages/V_F_measurements30 ==
  abc : Inport
  Display16 : Display
      settings: Format=bank
  PLL (3ph) : spsPLL3phLib/PLL (3ph)  Fmin=59.5  Par_Init=[0, 60]  ParK=[180, 3200, 1]  TcD=1e-4  MaxRateChangeFreq=12  FilterCutOffFreq=25  Ts=1e-5  AGC=on
  tag scope: f1=global, f_B30=global
  wires:
  abc/1 -> PLL (3ph)/1
  PLL (3ph)/1 -> [f1], [f_B30], Display16/1

== system Case3_IEEE39_UGFLandGFM_2022b/Bus voltages/V_F_measurements31 ==
  abc : Inport
  PLL (3ph) : spsPLL3phLib/PLL (3ph)  Fmin=59.5  Par_Init=[0, 60]  ParK=[180, 3200, 1]  TcD=1e-4  MaxRateChangeFreq=12  FilterCutOffFreq=25  Ts=1e-5  AGC=on
  tag scope: f2=global, f_B31=global
  wires:
  abc/1 -> PLL (3ph)/1
  PLL (3ph)/1 -> [f2], [f_B31]

== system Case3_IEEE39_UGFLandGFM_2022b/Bus voltages/V_F_measurements32 ==
  abc : Inport
  Display16 : Display
      settings: Format=bank
  PLL (3ph) : spsPLL3phLib/PLL (3ph)  Fmin=59.5  Par_Init=[0, 60]  ParK=[180, 3200, 1]  TcD=1e-4  MaxRateChangeFreq=12  FilterCutOffFreq=25  Ts=1e-5  AGC=on
  tag scope: f3=global, f_B32=global
  wires:
  abc/1 -> PLL (3ph)/1
  PLL (3ph)/1 -> [f3], [f_B32], Display16/1

== system Case3_IEEE39_UGFLandGFM_2022b/Bus voltages/V_F_measurements33 ==
  abc : Inport
  Display16 : Display
      settings: Format=bank
  PLL (3ph) : spsPLL3phLib/PLL (3ph)  Fmin=59.5  Par_Init=[0, 60]  ParK=[180, 3200, 1]  TcD=1e-4  MaxRateChangeFreq=12  FilterCutOffFreq=25  Ts=1e-5  AGC=on
  tag scope: f4=global, f_B33=global
  wires:
  abc/1 -> PLL (3ph)/1
  PLL (3ph)/1 -> [f_B33], Display16/1, [f4]

== system Case3_IEEE39_UGFLandGFM_2022b/Bus voltages/V_F_measurements34 ==
  abc : Inport
  Display16 : Display
      settings: Format=bank
  PLL (3ph) : spsPLL3phLib/PLL (3ph)  Fmin=59.5  Par_Init=[0, 60]  ParK=[180, 3200, 1]  TcD=1e-4  MaxRateChangeFreq=12  FilterCutOffFreq=25  Ts=1e-5  AGC=on
  tag scope: f5=global, f_B34=global
  wires:
  abc/1 -> PLL (3ph)/1
  PLL (3ph)/1 -> [f_B34], Display16/1, [f5]

== system Case3_IEEE39_UGFLandGFM_2022b/Bus voltages/V_F_measurements35 ==
  abc : Inport
  Display16 : Display
      settings: Format=bank
  PLL (3ph) : spsPLL3phLib/PLL (3ph)  Fmin=59.5  Par_Init=[0, 60]  ParK=[180, 3200, 1]  TcD=1e-4  MaxRateChangeFreq=12  FilterCutOffFreq=25  Ts=1e-5  AGC=on
  tag scope: f6=global, f_B35=global
  wires:
  abc/1 -> PLL (3ph)/1
  PLL (3ph)/1 -> [f6], [f_B35], Display16/1

== system Case3_IEEE39_UGFLandGFM_2022b/Bus voltages/V_F_measurements36 ==
  abc : Inport
  Display16 : Display
      settings: Format=bank
  PLL (3ph) : spsPLL3phLib/PLL (3ph)  Fmin=59.5  Par_Init=[0, 60]  ParK=[180, 3200, 1]  TcD=1e-4  MaxRateChangeFreq=12  FilterCutOffFreq=25  Ts=1e-5  AGC=on
  tag scope: f7=global, f_B36=global
  wires:
  abc/1 -> PLL (3ph)/1
  PLL (3ph)/1 -> [f7], [f_B36], Display16/1

== system Case3_IEEE39_UGFLandGFM_2022b/Bus voltages/V_F_measurements37 ==
  abc : Inport
  Display16 : Display
      settings: Format=bank
  PLL (3ph) : spsPLL3phLib/PLL (3ph)  Fmin=59.5  Par_Init=[0, 60]  ParK=[180, 3200, 1]  TcD=1e-4  MaxRateChangeFreq=12  FilterCutOffFreq=25  Ts=1e-5  AGC=on
  tag scope: f8=global, f_B37=global
  wires:
  abc/1 -> PLL (3ph)/1
  PLL (3ph)/1 -> [f8], [f_B37], Display16/1

== system Case3_IEEE39_UGFLandGFM_2022b/Bus voltages/V_F_measurements38 ==
  abc : Inport
  Display16 : Display
      settings: Format=bank
  PLL (3ph) : spsPLL3phLib/PLL (3ph)  Fmin=59.5  Par_Init=[0, 60]  ParK=[180, 3200, 1]  TcD=1e-4  MaxRateChangeFreq=12  FilterCutOffFreq=25  Ts=1e-5  AGC=on
  tag scope: f9=global, f_B38=global
  wires:
  abc/1 -> PLL (3ph)/1
  PLL (3ph)/1 -> [f9], [f_B38], Display16/1

== system Case3_IEEE39_UGFLandGFM_2022b/Bus voltages/V_F_measurements39 ==
  abc : Inport
  Display16 : Display
      settings: Format=bank
  PLL (3ph) : spsPLL3phLib/PLL (3ph)  Fmin=59.5  Par_Init=[0, 60]  ParK=[180, 3200, 1]  TcD=1e-4  MaxRateChangeFreq=12  FilterCutOffFreq=25  Ts=1e-5  AGC=on
  tag scope: f10=global, f_B39=global
  wires:
  abc/1 -> PLL (3ph)/1
  PLL (3ph)/1 -> [f10], [f_B39], Display16/1

== system Case3_IEEE39_UGFLandGFM_2022b/G3_GFL/PV_PQ3 ==
  Pref : Inport
  Qref : Inport  Port=2
  Fref : Inport  Port=3
  D : Inport  Port=4
  3-phase Instantaneous Active & Reactive Power4 : powerlib_extras/Measurements/3-phase  Instantaneous  Active & Reactive Power
  Controlled Voltage Source : spsControlledVoltageSourceLib/Controlled Voltage Source  Initialize=on  Source_Type=AC  Amplitude=391.87  Phase=0  Frequency=60  Measurements=None
  Controlled Voltage Source1 : spsControlledVoltageSourceLib/Controlled Voltage Source  Initialize=on  Source_Type=AC  Amplitude=391.87  Phase=-120  Frequency=60  Measurements=None
  Controlled Voltage Source3 : spsControlledVoltageSourceLib/Controlled Voltage Source  Initialize=on  Source_Type=AC  Amplitude=391.87  Phase=120  Frequency=60  Measurements=None
  Demux : Demux  Outputs=2
  Demux1 : Demux  Outputs=3
  Freq_Droop : Subsystem
  Gain2 : Gain  Gain=sqrt(3)/22000
  Ground : spsGroundLib/Ground  LConnTagsString=a
  Ground1 : spsGroundLib/Ground  LConnTagsString=a
  L : spsThreePhaseSeriesRLCBranchLib/Three-Phase Series RLC Branch  LConnTagsString=A|B|C  RConnTagsString=A|B|C  BranchType=RL  Resistance=0.01*Vbase^2/Sbase  Inductance=100e-3  Capacitance=1.0  Measurements=None
  L1 : Constant  Value=100e-3
  Mean : spsMeanLib/Mean  Freq=60  Vinit=0  Ts=1e-4
  PLL (3ph) : spsPLL3phLib/PLL (3ph)  Fmin=59.5  Par_Init=[0, 60]  ParK=[180, 3200, 1]  TcD=1e-4  MaxRateChangeFreq=12  FilterCutOffFreq=25  Ts=1e-5  AGC=on
  RMS Measurement : eeRmsMeasurement/RMS Measurement  LabelModeActiveChoice=Total  F=60  SpecifyHarmonics=off  K=[0 1 2]  Ts=1e-4
      settings: LibrarySourceBlock=|
      | ee_sl_lib/Measurements/RMS
      | Measurement
  Scope1 : Scope
  Scope5 : Scope
  Subsystem2 : Subsystem
  Terminator : Terminator
  Three-Phase Series RLC Branch : spsThreePhaseSeriesRLCBranchLib/Three-Phase Series RLC Branch  LConnTagsString=A|B|C  RConnTagsString=A|B|C  BranchType=RC  Resistance=1000000  Inductance=1e-3  Capacitance=10000e-6  Measurements=None
  Three-Phase V-I Measurement : spsThreePhaseVIMeasurementLib/Three-Phase V-I Measurement  VoltageMeasurement=phase-to-ground  SetLabelV=off  LabelV=Vabc  Vpu=off  VpuLL=off  CurrentMeasurement=yes  SetLabelI=off  LabelI=Iabc  Ipu=off  Pbase=1e5  Vbase=380  OutputType=Complex  PhasorSimulation=off  PSBequivalent=0
  Three-Phase V-I Measurement4 : spsThreePhaseVIMeasurementLib/Three-Phase V-I Measurement  VoltageMeasurement=phase-to-ground  SetLabelV=off  LabelV=u  Vpu=off  VpuLL=off  CurrentMeasurement=yes  SetLabelI=off  LabelI=iFabcp3  Ipu=off  Pbase=100e6  Vbase=500e3  OutputType=Complex  PhasorSimulation=off  PSBequivalent=0
  Unit Delay : UnitDelay  SampleTime=-1  HasFrameUpgradeWarning=on
  Unit Delay1 : UnitDelay  SampleTime=-1  HasFrameUpgradeWarning=on
  Unit Delay2 : UnitDelay  SampleTime=-1  HasFrameUpgradeWarning=on
  PV_BatteryA : PMIOPort  Side=Right
  PV_BatteryB : PMIOPort  Port=2  Side=Right
  PV_BatteryC : PMIOPort  Port=3  Side=Right
  tag scope: P_Bus32=global, Q_Bus32=global, V_Bus32=global
  wires:
  Three-Phase V-I Measurement/2 -> Subsystem2/2(Iabcp), 3-phase Instantaneous Active & Reactive Power4/2
  L1/1 -> Subsystem2/6(L1)
  Three-Phase V-I Measurement4/2 -> Subsystem2/3(IFabcp)
  3-phase Instantaneous Active & Reactive Power4/1 -> Mean/1
  Qref/1 -> Subsystem2/5(Q_set)
  Pref/1 -> Freq_Droop/1(Pref)
  Fref/1 -> Freq_Droop/2(Fref)
  [Freq] -> Freq_Droop/3(Freq)
  D/1 -> Freq_Droop/4(D)
  Freq_Droop/1(Pset) -> Subsystem2/4(P_set)
  Subsystem2/1(Va) -> Unit Delay/1
  Unit Delay/1 -> Controlled Voltage Source/1
  Subsystem2/2(Vb) -> Unit Delay1/1
  Unit Delay1/1 -> Controlled Voltage Source1/1
  Subsystem2/3(Vc) -> Unit Delay2/1
  Unit Delay2/1 -> Controlled Voltage Source3/1
  Demux/2 -> [Q_Bus32]
  Demux/1 -> [P_Bus32]
  Mean/1 -> Scope5/1, Demux/1
  PLL (3ph)/2 -> Terminator/1
  PLL (3ph)/1 -> [Freq]
  Three-Phase V-I Measurement4/1 -> Scope1/1
  RMS Measurement/1 -> Gain2/1
  Gain2/1 -> Demux1/1
  Three-Phase V-I Measurement/1 -> RMS Measurement/1, PLL (3ph)/1, 3-phase Instantaneous Active & Reactive Power4/1, Subsystem2/1(Vabcp)
  Demux1/1 -> [V_Bus32]
  connections:
  Three-Phase V-I Measurement/LConn1 -- Three-Phase Series RLC Branch/LConn1 -- L/RConn1
  Three-Phase V-I Measurement/RConn2 -- PV_BatteryB/RConn1
  Three-Phase V-I Measurement/LConn2 -- Three-Phase Series RLC Branch/LConn2 -- L/RConn2
  Three-Phase V-I Measurement4/LConn2 -- Controlled Voltage Source1/RConn1
  Controlled Voltage Source/RConn1 -- Three-Phase V-I Measurement4/LConn1
  Three-Phase V-I Measurement4/LConn3 -- Controlled Voltage Source3/RConn1
  Three-Phase V-I Measurement/LConn3 -- Three-Phase Series RLC Branch/LConn3 -- L/RConn3
  Three-Phase V-I Measurement/RConn3 -- PV_BatteryC/RConn1
  Three-Phase V-I Measurement/RConn1 -- PV_BatteryA/RConn1
  Three-Phase V-I Measurement4/RConn1 -- L/LConn1
  Three-Phase V-I Measurement4/RConn2 -- L/LConn2
  Three-Phase V-I Measurement4/RConn3 -- L/LConn3
  Three-Phase Series RLC Branch/RConn1 -- Ground1/LConn1 -- Three-Phase Series RLC Branch/RConn2 -- Three-Phase Series RLC Branch/RConn3
  Controlled Voltage Source/LConn1 -- Controlled Voltage Source3/LConn1 -- Controlled Voltage Source1/LConn1 -- Ground/LConn1

== system Case3_IEEE39_UGFLandGFM_2022b/GFM4/PV_PQ3 ==
  Pref : Inport
  Vref_LL : Inport  Port=2
  Fref : Inport  Port=3
  Initial_phase : Inport  Port=4
  3-phase Instantaneous Active & Reactive Power4 : powerlib_extras/Measurements/3-phase  Instantaneous  Active & Reactive Power
  Controlled Voltage Source : spsControlledVoltageSourceLib/Controlled Voltage Source  Initialize=on  Source_Type=DC  Amplitude=0  Phase=0  Frequency=60  Measurements=None
  Controlled Voltage Source1 : spsControlledVoltageSourceLib/Controlled Voltage Source  Initialize=on  Source_Type=DC  Amplitude=0  Phase=-120  Frequency=60  Measurements=None
  Controlled Voltage Source3 : spsControlledVoltageSourceLib/Controlled Voltage Source  Initialize=on  Source_Type=DC  Amplitude=0  Phase=120  Frequency=60  Measurements=None
  Demux : Demux  Outputs=2
  Demux1 : Demux  Outputs=3
  Freq_Droop : Subsystem
  Gain2 : Gain  Gain=sqrt(3)/22000
  Ground : spsGroundLib/Ground  LConnTagsString=a
  Ground1 : spsGroundLib/Ground  LConnTagsString=a
  L : spsThreePhaseSeriesRLCBranchLib/Three-Phase Series RLC Branch  LConnTagsString=A|B|C  RConnTagsString=A|B|C  BranchType=RL  Resistance=0.01*Vbase^2/Sbase  Inductance=0.08*Vbase^2/Sbase/377  Capacitance=1.0  Measurements=None
  Mean : spsMeanLib/Mean  Freq=60  Vinit=0  Ts=1e-2
  RMS Measurement : eeRmsMeasurement/RMS Measurement  LabelModeActiveChoice=Total  F=60  SpecifyHarmonics=off  K=[0 1 2]  Ts=1e-4
      settings: LibrarySourceBlock=|
      | ee_sl_lib/Measurements/RMS
      | Measurement
  Scope1 : Scope
  Scope2 : Scope
  Scope5 : Scope
  Three-Phase Series RLC Branch : spsThreePhaseSeriesRLCBranchLib/Three-Phase Series RLC Branch  LConnTagsString=A|B|C  RConnTagsString=A|B|C  BranchType=C  Resistance=0  Inductance=1e-3  Capacitance=1e-6  Measurements=None
  Three-Phase V-I Measurement : spsThreePhaseVIMeasurementLib/Three-Phase V-I Measurement  VoltageMeasurement=phase-to-ground  SetLabelV=off  LabelV=Vabc  Vpu=off  VpuLL=off  CurrentMeasurement=yes  SetLabelI=off  LabelI=Iabc  Ipu=off  Pbase=1e5  Vbase=380  OutputType=Complex  PhasorSimulation=off  PSBequivalent=0
  Three-Phase V-I Measurement4 : spsThreePhaseVIMeasurementLib/Three-Phase V-I Measurement  VoltageMeasurement=no  SetLabelV=off  LabelV=u  Vpu=off  VpuLL=off  CurrentMeasurement=yes  SetLabelI=off  LabelI=iFabcp3  Ipu=off  Pbase=100e6  Vbase=500e3  OutputType=Complex  PhasorSimulation=off  PSBequivalent=0
  Unit Delay : UnitDelay  SampleTime=-1  HasFrameUpgradeWarning=on
  Unit Delay1 : UnitDelay  SampleTime=-1  HasFrameUpgradeWarning=on
  Unit Delay2 : UnitDelay  SampleTime=-1  HasFrameUpgradeWarning=on
  V/F : Subsystem
  PV_BatteryA : PMIOPort  Side=Right
  PV_BatteryB : PMIOPort  Port=2  Side=Right
  PV_BatteryC : PMIOPort  Port=3  Side=Right
  tag scope: P_Bus31=global, Q_Bus31=global, V_Bus31=global
  wires:
  Three-Phase V-I Measurement/2 -> V/F/2(iabcb), Scope2/1, 3-phase Instantaneous Active & Reactive Power4/2
  Mean/1 -> Scope5/1, Demux/1
  Three-Phase V-I Measurement4/1 -> V/F/3(iFabcb)
  3-phase Instantaneous Active & Reactive Power4/1 -> Mean/1
  Pref/1 -> Freq_Droop/1(Pref)
  Fref/1 -> Freq_Droop/2(Fref)
  [P_meas] -> Freq_Droop/3(Pmeans)
  Freq_Droop/1(fset) -> V/F/5(f)
  Vref_LL/1 -> V/F/4(Vref_LL)
  Initial_phase/1 -> V/F/6(Init_Phase_degree)
  Unit Delay/1 -> Controlled Voltage Source/1
  V/F/1(Va) -> Unit Delay/1
  Unit Delay1/1 -> Controlled Voltage Source1/1
  V/F/2(Vb) -> Unit Delay1/1
  Unit Delay2/1 -> Controlled Voltage Source3/1
  V/F/3(Vc) -> Unit Delay2/1
  Demux/1 -> [P_Bus31], [P_meas]
  Three-Phase V-I Measurement/1 -> RMS Measurement/1, 3-phase Instantaneous Active & Reactive Power4/1, Scope1/1, V/F/1(vabcb)
  RMS Measurement/1 -> Gain2/1
  Gain2/1 -> Demux1/1
  Demux1/1 -> [V_Bus31]
  Demux/2 -> [Q_Bus31]
  connections:
  Three-Phase V-I Measurement/LConn1 -- Three-Phase Series RLC Branch/LConn1 -- L/RConn1
  Three-Phase V-I Measurement/RConn2 -- PV_BatteryB/RConn1
  Three-Phase V-I Measurement/LConn2 -- Three-Phase Series RLC Branch/LConn2 -- L/RConn2
  Three-Phase V-I Measurement4/LConn2 -- Controlled Voltage Source1/RConn1
  Controlled Voltage Source/RConn1 -- Three-Phase V-I Measurement4/LConn1
  Three-Phase V-I Measurement4/LConn3 -- Controlled Voltage Source3/RConn1
  Three-Phase V-I Measurement/LConn3 -- Three-Phase Series RLC Branch/LConn3 -- L/RConn3
  Three-Phase V-I Measurement/RConn3 -- PV_BatteryC/RConn1
  Three-Phase V-I Measurement/RConn1 -- PV_BatteryA/RConn1
  Three-Phase V-I Measurement4/RConn1 -- L/LConn1
  Three-Phase V-I Measurement4/RConn2 -- L/LConn2
  Three-Phase V-I Measurement4/RConn3 -- L/LConn3
  Three-Phase Series RLC Branch/RConn1 -- Ground1/LConn1 -- Three-Phase Series RLC Branch/RConn2 -- Three-Phase Series RLC Branch/RConn3
  Controlled Voltage Source/LConn1 -- Controlled Voltage Source3/LConn1 -- Controlled Voltage Source1/LConn1 -- Ground/LConn1
